simulink model "ssc_dcmotor"  (R2013a)
settings: Solver=ode15s  StartTime=0.0  StopTime=0.2  MaxStep=0.001  RelTol=1e-3
libraries: fl_lib x12, nesl_utility x4
Description:
  | Permanent Magnet DC Motor
  | 
  | This model is based on a Faulhaber Series 0615 DC-Micromotor. For the 1.5V
  | variant, equivalent circuit parameters are given as:
  | 
  |   Rotor resistance R=3.9 Ohms
  |   Rotor inductance L=12uH
  |   Back emf constant K=0.072mV/rpm
  |   Rotor inertia J=0.01gcm^2
  |   Friction torque Mr=0.02mNm
  | 
  | The model uses these parameters to verify manufacturer-quoted no-load speed,
  | no-load current, and stall torque, which are:
  | 
  |   No-load speed = 19,100rpm
  |   No-load current = 0.03A
  |   Stall torque = 0.24mNm
  | 
  | When running the simulation, for the first 0.1 seconds the motor  has no external
  | load, and the speed builds up to the no-load value. Then at 0.1 seconds the stall
  | torque is applied as a load to the motor shaft. Zooming in on the RPM and Motor
  | Current scopes shows a good level of agreement with manufacturer data.
  | 
  | Often manufacturers do not quote the equivalent circuit parameters, and they must
  | be estimated from information such as no-load speed, stall torque, and efficiency.
  | A test harness such as this model can then be used to test the estimated
  | equivalent circuit prior to using the motor model in a complete system simulation.
  | 
  | 
  | Copyright 2008-2013 The MathWorks, Inc.
settings Model: ExtModeAutoUpdateStatusClock=off  Creator=MathWorks  LastModifiedBy=mainster
settings DataIOCC: SignalLoggingSaveFormat=ModelDataLogs
settings OptimizationCC: ExpressionDepthLimit=2147483647  InitFltsAndDblsToZero=on
settings DebuggingCC: SaveWithParameterizedLinksMsg=none  SignalResolutionControl=TryResolveAllWithWarning  FcnCallInpInsideContextMsg=UseLocalSettings  StrictBusMsg=Warning
settings GRTTargetCC: TargetFcnLib=ansi_tfl_tmw.mat  CombineOutputUpdateFcns=off  GRTInterface=on

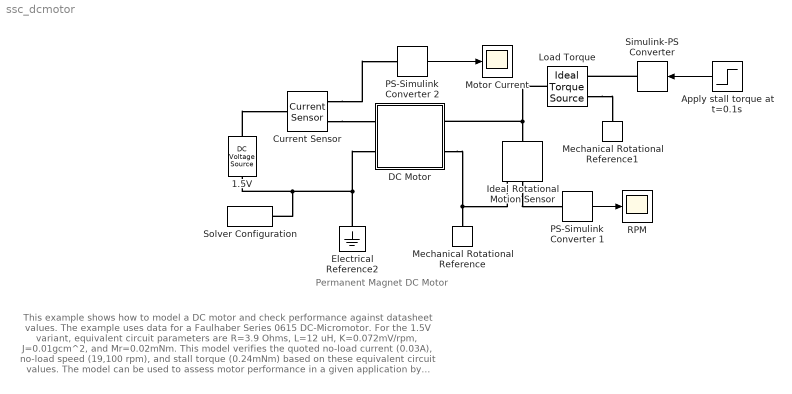
== system ssc_dcmotor ==
  note: This example shows how to model a DC motor and check performance
      | against datasheet values. The example uses data for a Faulhaber
      | Series  0615 DC-Micromotor. For the 1.5V variant, equivalent circuit
      | parameters are R=3.9 Ohms, L=12 uH, K=0.072mV/rpm, J=0.01gcm^2,
      | and Mr=0.02mNm. This model verifies the quoted no-load current
      | (0.03A), no-load speed (19,100 rpm), and stall torque (0.24mNm)
      | based on these equivalent circuit values. The model can be used to
      | assess motor performance in a given application by adding the
      | requisite mechanical load model.
  note: Permanent Magnet DC Motor
  1.5V : fl_lib/Electrical/Electrical Sources/DC Voltage Source  v0=1.5 V  i_Log=off  v_Log=off  LocalVarNames=|current|voltage|power  LocalVarDescs=|Current (A)|Voltage (V)|Power (W)  LocalVarLogging=[0 0 0]
  Apply stall torque at t=0.1s : Step  Time=0.1  After=-0.24e-3  SampleTime=0
  Current Sensor : fl_lib/Electrical/Electrical Sensors/Current Sensor  i1_Log=off  v1_Log=off  LocalVarNames=|i1|v1  LocalVarDescs=|i1|v1  LocalVarLogging=[]
  DC Motor : Subsystem
  Electrical Reference2 : fl_lib/Electrical/Electrical Elements/Electrical Reference  i_Log=off  LocalVarNames=|i  LocalVarDescs=|i  LocalVarLogging=[]
  Ideal Rotational Motion Sensor : fl_lib/Mechanical/Mechanical Sensors/Ideal Rotational Motion Sensor  offset=0 rad  w_Log=off  t_Log=off  phi_Log=off  LocalVarNames=|w|t|phi  LocalVarDescs=|w|t|phi  LocalVarLogging=[]
  Load Torque : fl_lib/Mechanical/Mechanical Sources/Ideal Torque Source  w_Log=off  t_Log=off  LocalVarNames=|torque|rel_velocity|power  LocalVarDescs=|Torque (N*m)|Relative velocity (rad/s)|Power generated by the source (W)  LocalVarLogging=[0 0 0]
  Mechanical Rotational Reference : fl_lib/Mechanical/Rotational Elements/Mechanical Rotational Reference  t_Log=off  LocalVarNames=|t  LocalVarDescs=|t  LocalVarLogging=[]
  Mechanical Rotational Reference1 : fl_lib/Mechanical/Rotational Elements/Mechanical Rotational Reference  t_Log=off  LocalVarNames=|t  LocalVarDescs=|t  LocalVarLogging=[]
  Motor Current : Scope
      settings: YMin=-1  YMax=1
  PS-Simulink Converter 1 : nesl_utility/PS-Simulink Converter  PhysicalDomain=network_engine_domain  SubClassName=ps_output  LeftPortType=input  RightPortType=output  PseudoPeriodic=off  Frequencies=[]  Unit=rpm  AffineConversion=off
  PS-Simulink Converter 2 : nesl_utility/PS-Simulink Converter  PhysicalDomain=network_engine_domain  SubClassName=ps_output  LeftPortType=input  RightPortType=output  PseudoPeriodic=off  Frequencies=[]  Unit=1  AffineConversion=off
  RPM : Scope
      settings: YMin=0  YMax=20000
  Simulink-PS Converter : nesl_utility/Simulink-PS Converter  PhysicalDomain=network_engine_domain  SubClassName=ps_input  LeftPortType=input  RightPortType=output  PseudoPeriodic=off  Frequencies=[]  NoiseDistribution=none  NoiseParameters=[]  Unit=1  AffineConversion=off  InputFiltering=off  SimscapeFilterOrder=1  InputFilterTimeConstant=.001  UdotUserProvided=0
  Solver Configuration : nesl_utility/Solver Configuration  PhysicalDomain=network_engine_domain  SubClassName=solver  LeftPortType=input  RightPortType=generic  Accelerate=off  Tones=[]  Harmonics=[]  SimulateNoise=off  Profile=off  UseLocalSampling=off  EnableSwitchedLinearOptims=on  FrequencyDomain=off  UseCCode=off  UseNewInitialization=off  DoDC=off  ResidualTolerance=1e-9  UseLocalSolver=off  LocalSolverChoice=NE_BACKWARD_EULER_ADVANCER  LocalSolverSampleTime=.001  DoFixedCost=off  MaxNonlinIter=3  MaxModeIter=2  LinearAlgebra=Sparse  DelaysMemoryBudget=1024
  wires:
  PS-Simulink Converter 1/1 -> RPM/1
  PS-Simulink Converter 2/1 -> Motor Current/1
  Apply stall torque at t=0.1s/1 -> Simulink-PS Converter/1
  connections:
  DC Motor/LConn2 -- Electrical Reference2/LConn1 -- 1.5V/RConn1 -- Solver Configuration/RConn1
  1.5V/LConn1 -- Current Sensor/LConn1
  Current Sensor/RConn2 -- DC Motor/LConn1
  Current Sensor/RConn1 -- PS-Simulink Converter 2/LConn1
  DC Motor/RConn2 -- Mechanical Rotational Reference/LConn1 -- Ideal Rotational Motion Sensor/RConn1
  Load Torque/LConn1 -- DC Motor/RConn1 -- Ideal Rotational Motion Sensor/LConn1
  Ideal Rotational Motion Sensor/RConn2 -- PS-Simulink Converter 1/LConn1
  Load Torque/RConn2 -- Mechanical Rotational Reference1/LConn1
  Simulink-PS Converter/RConn1 -- Load Torque/RConn1

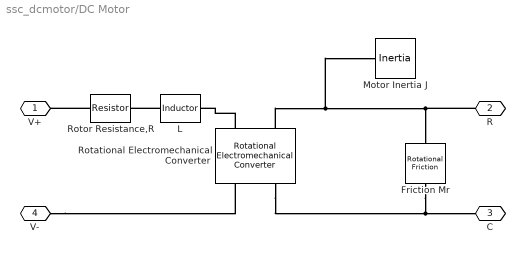
== system ssc_dcmotor/DC Motor ==
  Friction Mr : fl_lib/Mechanical/Rotational Elements/Rotational Friction  brkwy_trq=0.02e-3 N*m  Col_trq=0.02e-3 N*m  visc_coef=0 N*m/(rad/s)  trans_coef=10 s/rad  vel_thr=0.1 rad/s  t_Log=off  w_Log=off  LocalVarNames=|friction_torque|rel_velocity|power  LocalVarDescs=|Friction torque (N*m)|Relative velocity (rad/s)|Power (W)  LocalVarLogging=[0 0 0]
  L : fl_lib/Electrical/Electrical Elements/Inductor  l=12e-6 H  i0=0 A  r=0 Ohm  g=1e-09 1/Ohm  i_Log=off  v_Log=off  i_L_Log=off  LocalVarNames=|current|voltage|power  LocalVarDescs=|Inductor current (A) |Voltage across inductor (V)|Power (W)  LocalVarLogging=[0 0 0]
  Motor Inertia J : fl_lib/Mechanical/Rotational Elements/Inertia  inertia=0.01 g*cm^2  initial_velocity=0 rad/s  t_Log=off  LocalVarNames=|torque|velocity  LocalVarDescs=|Inertia torque (N*m)|Inertia absolute velocity (rad/s)  LocalVarLogging=[0 0]
  Rotational Electromechanical Converter : fl_lib/Electrical/Electrical Elements/Rotational Electromechanical Converter  K=0.072e-3*60/(2*pi) s*V/rad  i_Log=off  v_Log=off  t_Log=off  w_Log=off  LocalVarNames=|current|voltage|power|torque|speed  LocalVarDescs=|Current (A)|Voltage (V)|Power (W)|Torque (Nm)|Angular speed (rad/s)  LocalVarLogging=[0 0 0 0 0]
  Rotor Resistance,R : fl_lib/Electrical/Electrical Elements/Resistor  Tag=Factory Generic  R=3.9 Ohm  i_Log=off  v_Log=off  LocalVarNames=|current|voltage|power  LocalVarDescs=|Resistor current (A)|Voltage across resistor (V)|Power (W)  LocalVarLogging=[0 0 0]
  V+ : PMIOPort  Port=1  Side=Left
  R : PMIOPort  Port=2  Side=Right
  C : PMIOPort  Port=3  Side=Right
  V- : PMIOPort  Port=4  Side=Left
  connections:
  Rotational Electromechanical Converter/LConn1 -- L/RConn1
  V-/RConn1 -- Rotational Electromechanical Converter/RConn1
  Rotor Resistance,R/LConn1 -- V+/RConn1
  L/LConn1 -- Rotor Resistance,R/RConn1
  Rotational Electromechanical Converter/LConn2 -- R/RConn1 -- Friction Mr/LConn1 -- Motor Inertia J/LConn1
  Rotational Electromechanical Converter/RConn2 -- C/RConn1 -- Friction Mr/RConn1
